simulink model "SimulinkModelisation"  (R2016b)
settings: Solver=VariableStepAuto  StartTime=0.0  StopTime=10.0  RelTol=1e-3  EnableMultiTasking=on
values from neighbouring files (symbols this model uses):
  A = [line1;line2;line3;line4;line5]    [sm_7.m]
  B = [m0_3x3; m0_3x3; m0_2x3; m0_2x3; mCV_3x3]    [sm_7.m]
  C = [mTTdef m0_3x3 m0_3x4 m0_3x3 ... (first row only)    [sm_7.m]
  D = zeros(7,3)    [sm_7.m]
undefined symbols (not defined in the file or in its folder): ae0, ae1, ae2, ae3, as0, as1, as2, as3, be1, C_prime, D_prime, ia_e, ib_e, ic_e, phi_e, TABC_trans, TDEF_trans, theta_e, va_e, vb_e, vc_e, vx_s_e, vy_s_e, vz_e, w_phi_e, w_theta_e, x_s_e, y_s_e, z_e, za_e, zb_e, zc_e, zd_e, ze_e, zf_e
settings Model: Creator=JayMcGee  LastModifiedBy=Sytten
settings OptimizationCC: LifeSpan=inf
settings DebuggingCC: SFUnexpectedBacktrackingDiag=warning  SFNoUnconditionalDefaultTransitionDiag=warning  SFExecutionAtInitializationDiag=none
settings GRTTargetCC: TargetLangStandard=C89/C90 (ANSI)  GeneratePreprocessorConditionals=Disable all
settings ConfigComp: CovMetricSettings=dw  CovHtmlReporting=on  CovSaveCumulativeToWorkspaceVar=on  CovSaveSingleToWorkspaceVar=on  CovExternalEMLEnable=off

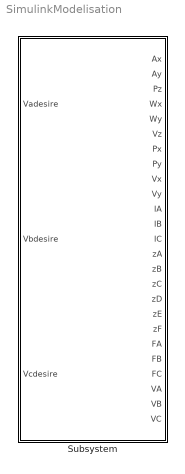
== system SimulinkModelisation ==
  Subsystem : Subsystem

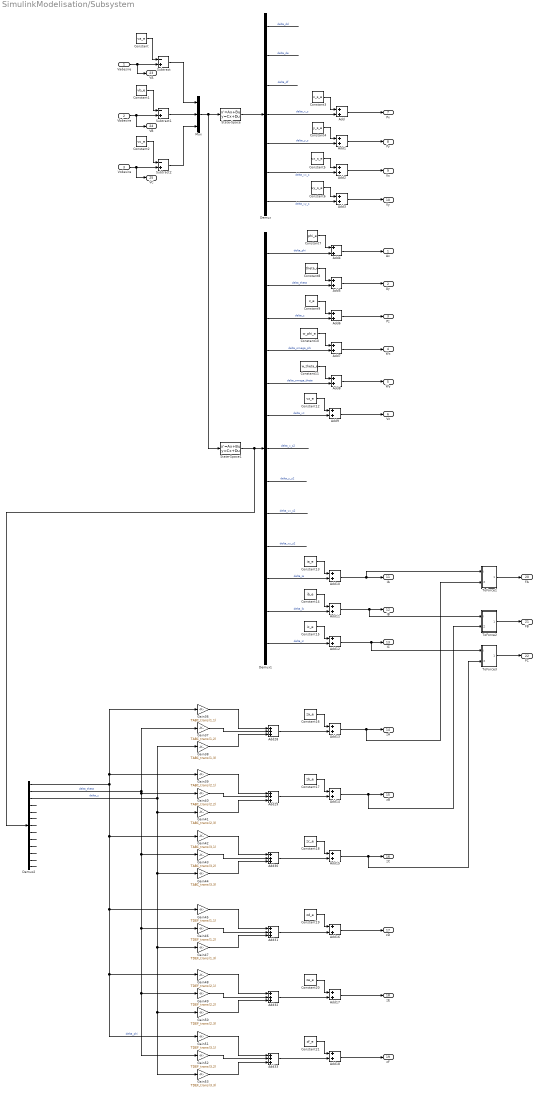
== system SimulinkModelisation/Subsystem ==
  Vadesire : Inport
  Vbdesire : Inport  Port=2
  Vcdesire : Inport  Port=3
  Add{,1..18} (19 alike) : Sum
  Add{28..33} (6 alike) : Sum  Inputs=+++
  Constant : Constant  Value=va_e
  Constant1 : Constant  Value=vb_e
  Constant10 : Constant  Value=w_phi_e
  Constant11 : Constant  Value=w_theta_e
  Constant12 : Constant  Value=vz_e
  Constant13 : Constant  Value=ia_e
  Constant14 : Constant  Value=ib_e
  Constant15 : Constant  Value=ic_e
  Constant16 : Constant  Value=za_e
  Constant17 : Constant  Value=zb_e
  Constant18 : Constant  Value=zc_e
  Constant19 : Constant  Value=zd_e
  Constant2 : Constant  Value=vc_e
  Constant20 : Constant  Value=ze_e
  Constant21 : Constant  Value=zf_e
  Constant3 : Constant  Value=x_s_e
  Constant4 : Constant  Value=y_s_e
  Constant5 : Constant  Value=vx_s_e
  Constant6 : Constant  Value=vy_s_e
  Constant7 : Constant  Value=phi_e
  Constant8 : Constant  Value=theta_e
  Constant9 : Constant  Value=z_e
  Demux : Demux  Outputs=7
  Demux1 : Demux  Outputs=13
  Demux2 : Demux  Outputs=13
  Gain36 : Gain  Gain=TABC_trans(1,1)
  Gain37 : Gain  Gain=TABC_trans(1,2)
  Gain38 : Gain  Gain=TABC_trans(1,3)
  Gain39 : Gain  Gain=TABC_trans(2,1)
  Gain40 : Gain  Gain=TABC_trans(2,2)
  Gain41 : Gain  Gain=TABC_trans(2,3)
  Gain42 : Gain  Gain=TABC_trans(3,1)
  Gain43 : Gain  Gain=TABC_trans(3,2)
  Gain44 : Gain  Gain=TABC_trans(3,3)
  Gain45 : Gain  Gain=TDEF_trans(1,1)
  Gain46 : Gain  Gain=TDEF_trans(1,2)
  Gain47 : Gain  Gain=TDEF_trans(1,3)
  Gain48 : Gain  Gain=TDEF_trans(2,1)
  Gain49 : Gain  Gain=TDEF_trans(2,2)
  Gain50 : Gain  Gain=TDEF_trans(2,3)
  Gain51 : Gain  Gain=TDEF_trans(3,1)
  Gain52 : Gain  Gain=TDEF_trans(3,2)
  Gain53 : Gain  Gain=TDEF_trans(3,3)
  Mux : Mux  Inputs=3
  State-Space : StateSpace  A=A  B=B  C=C  D=D  X0=0
  State-Space1 : StateSpace  A=A  B=B  C=C_prime  D=D_prime  X0=0
  Subtract : Sum  Inputs=-+
  Subtract1 : Sum  Inputs=-+
  Subtract2 : Sum  Inputs=-+
  ToForce1 : Subsystem
  ToForce2 : Subsystem
  ToForce3 : Subsystem
  Ax : Outport
  Ay : Outport  Port=2
  Pz : Outport  Port=3
  Wx : Outport  Port=4
  Wy : Outport  Port=5
  Vz : Outport  Port=6
  Px : Outport  Port=7
  Py : Outport  Port=8
  Vx : Outport  Port=9
  Vy : Outport  Port=10
  IA : Outport  Port=11
  IB : Outport  Port=12
  IC : Outport  Port=13
  zA : Outport  Port=14
  zB : Outport  Port=15
  zC : Outport  Port=16
  zD : Outport  Port=17
  zE : Outport  Port=18
  zF : Outport  Port=19
  FA : Outport  Port=20
  FB : Outport  Port=21
  FC : Outport  Port=22
  VA : Outport  Port=23
  VB : Outport  Port=24
  VC : Outport  Port=25
  wires:
  Demux2/6 -> ?
  Demux2/11 -> ?
  Add11/1 -> ToForce2/1(I), IB/1
  Demux2/7 -> ?
  Demux2/13 -> ?
  Gain44/1 -> Add30/3
  Constant13/1 -> Add10/1
  Constant15/1 -> Add12/1
  Gain50/1 -> Add32/3
  Demux1/13 -> Add12/2  "delta_ic"
  Demux1/7 -> ?  "delta_x_s2"
  Gain52/1 -> Add33/2
  Gain36/1 -> Add28/1
  Constant14/1 -> Add11/1
  Demux2/1 -> Gain48/1, Gain51/1, Gain45/1, Gain42/1, Gain39/1, Gain36/1  "delta_phi"
  Gain38/1 -> Add28/3
  Demux2/2 -> Gain37/1, Gain40/1, Gain52/1, Gain49/1, Gain46/1, Gain43/1  "delta_theta"
  Constant18/1 -> Add15/1
  Add28/1 -> Add13/2
  Add29/1 -> Add14/2
  Demux1/1 -> Add4/2  "delta_phi"
  Gain39/1 -> Add29/1
  Constant16/1 -> Add13/1
  Add30/1 -> Add15/2
  Constant11/1 -> Add8/1
  Demux1/4 -> Add7/2  "delta_omega_phi"
  Add2/1 -> Vx/1
  State-Space1/1 -> Demux2/1, Demux1/1
  Constant1/1 -> Subtract1/1
  Add1/1 -> Py/1
  Demux/2 -> ?  "delta_de"
  Vadesire/1 -> VA/1, Subtract/2
  Add3/1 -> Vy/1
  Constant17/1 -> Add14/1
  Constant4/1 -> Add1/1
  Constant3/1 -> Add/1
  Demux/4 -> Add/2  "delta_x_s"
  Demux/3 -> ?  "delta_df"
  Add9/1 -> Vz/1
  Constant12/1 -> Add9/1
  Constant5/1 -> Add2/1
  Demux1/6 -> Add9/2  "delta_vz"
  Demux1/10 -> ?  "delta_vy_s2"
  Vcdesire/1 -> VC/1, Subtract2/2
  Subtract1/1 -> Mux/2
  Add8/1 -> Wy/1
  Constant2/1 -> Subtract2/1
  Constant6/1 -> Add3/1
  Subtract2/1 -> Mux/3
  Add16/1 -> zD/1
  Add17/1 -> zE/1
  State-Space/1 -> Demux/1
  Gain53/1 -> Add33/3
  Demux1/9 -> ?  "delta_vx_s2"
  Demux2/10 -> ?
  Add33/1 -> Add18/2
  Demux/1 -> ?  "delta_dd"
  Subtract/1 -> Mux/1
  Demux/5 -> Add1/2  "delta_y_s"
  Add13/1 -> ToForce1/2(Z), zA/1
  Gain48/1 -> Add32/1
  Gain51/1 -> Add33/1
  Add15/1 -> ToForce3/2(Z), zC/1
  Add7/1 -> Wx/1
  Gain47/1 -> Add31/3
  Add14/1 -> ToForce2/2(Z), zB/1
  Constant10/1 -> Add7/1
  Add18/1 -> zF/1
  Gain43/1 -> Add30/2
  Demux2/3 -> Gain53/1, Gain50/1, Gain47/1, Gain44/1, Gain41/1, Gain38/1  "delta_z"
  Constant/1 -> Subtract/1
  Constant19/1 -> Add16/1
  Add32/1 -> Add17/2
  Add31/1 -> Add16/2
  Gain42/1 -> Add30/1
  Gain41/1 -> Add29/3
  Demux1/2 -> Add5/2  "delta_theta"
  Gain49/1 -> Add32/2
  Mux/1 -> State-Space1/1, State-Space/1
  Demux1/8 -> ?  "delta_y_s2"
  Demux/7 -> Add3/2  "delta_vy_s"
  Constant20/1 -> Add17/1
  Gain40/1 -> Add29/2
  Demux1/5 -> Add8/2  "delta_omega_theta"
  Demux2/4 -> ?
  Demux2/9 -> ?
  Demux2/8 -> ?
  Demux2/5 -> ?
  Demux1/12 -> Add11/2  "delta_ib"
  Vbdesire/1 -> VB/1, Subtract1/2
  Add/1 -> Px/1
  Demux/6 -> Add2/2  "delta_vx_s"
  Gain37/1 -> Add28/2
  Constant7/1 -> Add4/1
  Constant9/1 -> Add6/1
  Add5/1 -> Ay/1
  Add12/1 -> ToForce3/1(I), IC/1
  Demux1/3 -> Add6/2  "delta_z"
  Add6/1 -> Pz/1
  Constant8/1 -> Add5/1
  Gain46/1 -> Add31/2
  Demux1/11 -> Add10/2  "delta_ia"
  Gain45/1 -> Add31/1
  Add4/1 -> Ax/1
  Add10/1 -> ToForce1/1(I), IA/1
  Constant21/1 -> Add18/1
  Demux2/12 -> ?
  ToForce1/1(Force) -> FA/1
  ToForce2/1(Force) -> FB/1
  ToForce3/1(Force) -> FC/1

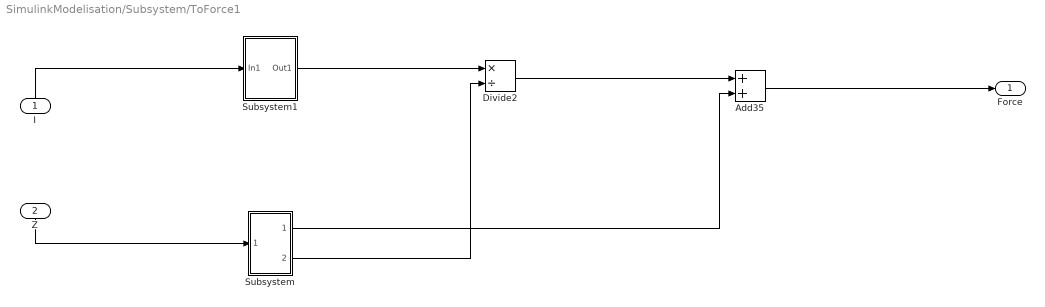
== system SimulinkModelisation/Subsystem/ToForce1 ==
  I : Inport
  Z : Inport  Port=2
  Add35 : Sum
  Divide2 : Product  Inputs=*/
  Subsystem : Subsystem
  Subsystem1 : Subsystem
  Force : Outport
  wires:
  Subsystem1/1(Out1) -> Divide2/1
  Z/1 -> Subsystem/1(In1)
  Subsystem/2(Out2) -> Divide2/2
  Divide2/1 -> Add35/1
  Add35/1 -> Force/1
  I/1 -> Subsystem1/1(In1)
  Subsystem/1(Out1) -> Add35/2

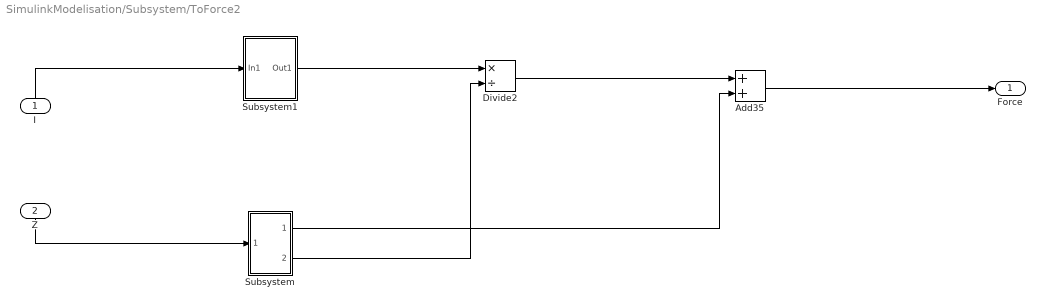
== system SimulinkModelisation/Subsystem/ToForce2 ==
  I : Inport
  Z : Inport  Port=2
  Add35 : Sum
  Divide2 : Product  Inputs=*/
  Subsystem : Subsystem
  Subsystem1 : Subsystem
  Force : Outport
  wires:
  Subsystem1/1(Out1) -> Divide2/1
  Z/1 -> Subsystem/1(In1)
  Subsystem/2(Out2) -> Divide2/2
  Divide2/1 -> Add35/1
  Add35/1 -> Force/1
  I/1 -> Subsystem1/1(In1)
  Subsystem/1(Out1) -> Add35/2

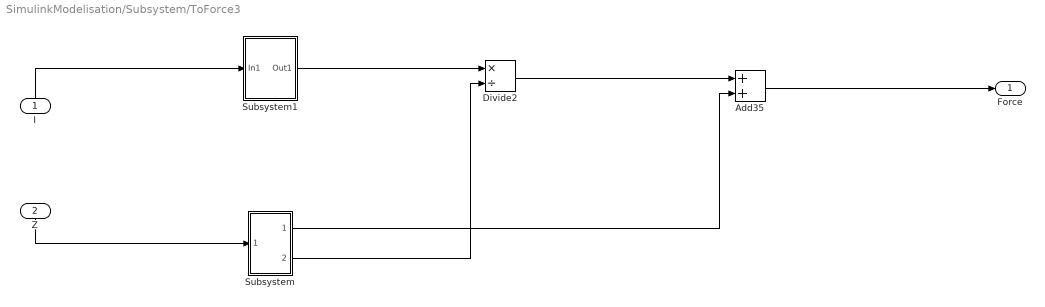
== system SimulinkModelisation/Subsystem/ToForce3 ==
  I : Inport
  Z : Inport  Port=2
  Add35 : Sum
  Divide2 : Product  Inputs=*/
  Subsystem : Subsystem
  Subsystem1 : Subsystem
  Force : Outport
  wires:
  Subsystem1/1(Out1) -> Divide2/1
  Z/1 -> Subsystem/1(In1)
  Subsystem/2(Out2) -> Divide2/2
  Divide2/1 -> Add35/1
  Add35/1 -> Force/1
  I/1 -> Subsystem1/1(In1)
  Subsystem/1(Out1) -> Add35/2

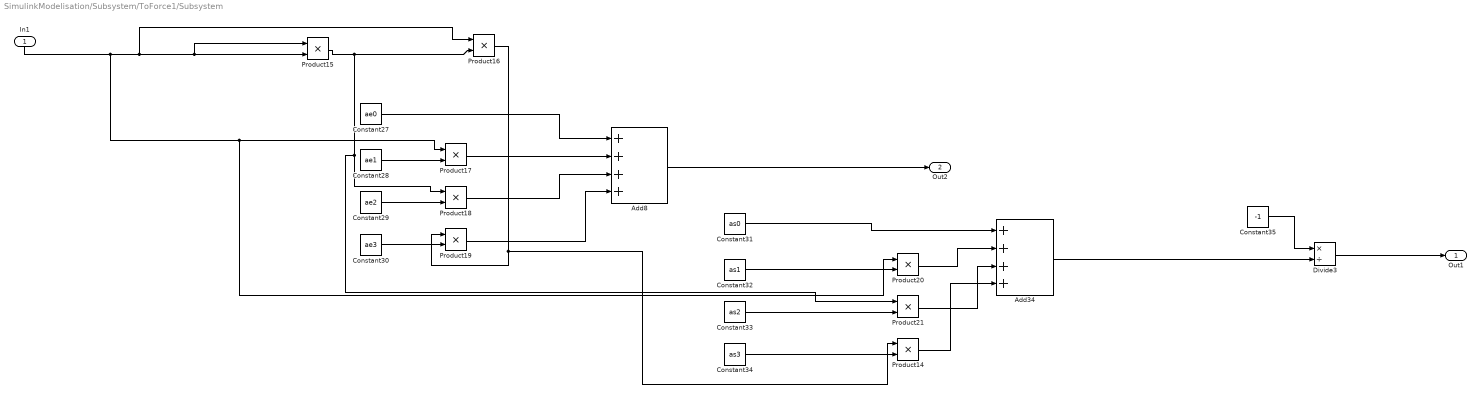
== system SimulinkModelisation/Subsystem/ToForce1/Subsystem ==
  In1 : Inport
  Add34 : Sum  Inputs=++++
  Add8 : Sum  Inputs=++++
  Constant27 : Constant  Value=ae0
  Constant28 : Constant  Value=ae1
  Constant29 : Constant  Value=ae2
  Constant30 : Constant  Value=ae3
  Constant31 : Constant  Value=as0
  Constant32 : Constant  Value=as1
  Constant33 : Constant  Value=as2
  Constant34 : Constant  Value=as3
  Constant35 : Constant  Value=-1
  Divide3 : Product  Inputs=*/
  Product{14..21} (8 alike) : Product
  Out1 : Outport
  Out2 : Outport  Port=2
  wires:
  In1/1 -> Product20/1, Product17/1, Product16/1, Product15/1, Product15/2
  Constant28/1 -> Product17/2
  Constant30/1 -> Product19/2
  Constant29/1 -> Product18/2
  Product15/1 -> Product21/1, Product18/1, Product16/2
  Product16/1 -> Product19/1, Product14/1
  Constant27/1 -> Add8/1
  Product17/1 -> Add8/2
  Product18/1 -> Add8/3
  Product19/1 -> Add8/4
  Add8/1 -> Out2/1
  Constant34/1 -> Product14/2
  Constant32/1 -> Product20/2
  Constant33/1 -> Product21/2
  Product20/1 -> Add34/2
  Product21/1 -> Add34/3
  Product14/1 -> Add34/4
  Constant31/1 -> Add34/1
  Add34/1 -> Divide3/2
  Constant35/1 -> Divide3/1
  Divide3/1 -> Out1/1

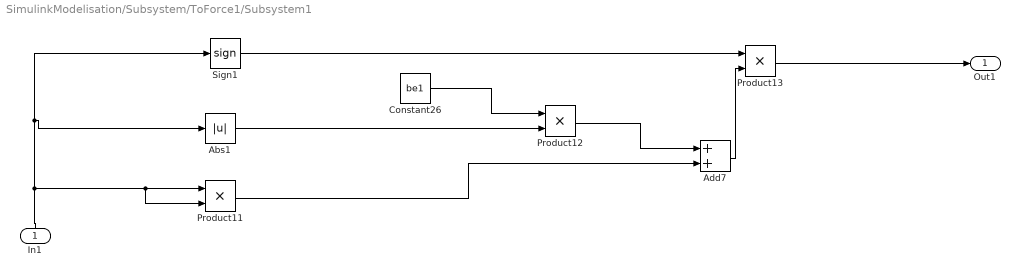
== system SimulinkModelisation/Subsystem/ToForce1/Subsystem1 ==
  In1 : Inport
  Abs1 : Abs
  Add7 : Sum
  Constant26 : Constant  Value=be1
  Product11 : Product
  Product12 : Product
  Product13 : Product
  Sign1 : Signum
  Out1 : Outport
  wires:
  In1/1 -> Abs1/1, Sign1/1, Product11/2, Product11/1
  Constant26/1 -> Product12/1
  Abs1/1 -> Product12/2
  Product12/1 -> Add7/1
  Product11/1 -> Add7/2
  Add7/1 -> Product13/2
  Product13/1 -> Out1/1
  Sign1/1 -> Product13/1

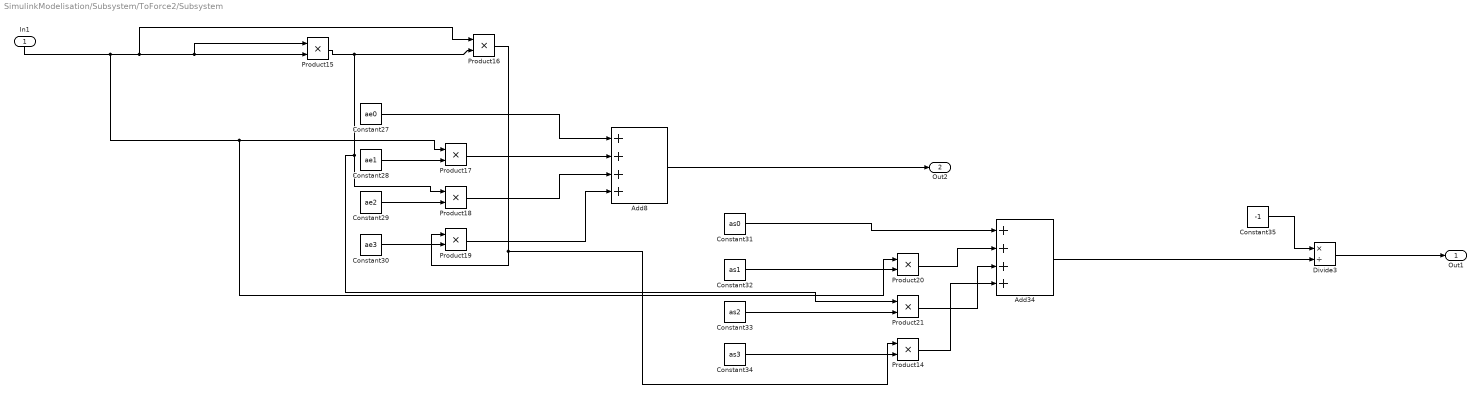
== system SimulinkModelisation/Subsystem/ToForce2/Subsystem ==
  In1 : Inport
  Add34 : Sum  Inputs=++++
  Add8 : Sum  Inputs=++++
  Constant27 : Constant  Value=ae0
  Constant28 : Constant  Value=ae1
  Constant29 : Constant  Value=ae2
  Constant30 : Constant  Value=ae3
  Constant31 : Constant  Value=as0
  Constant32 : Constant  Value=as1
  Constant33 : Constant  Value=as2
  Constant34 : Constant  Value=as3
  Constant35 : Constant  Value=-1
  Divide3 : Product  Inputs=*/
  Product{14..21} (8 alike) : Product
  Out1 : Outport
  Out2 : Outport  Port=2
  wires:
  In1/1 -> Product20/1, Product17/1, Product16/1, Product15/1, Product15/2
  Constant28/1 -> Product17/2
  Constant30/1 -> Product19/2
  Constant29/1 -> Product18/2
  Product15/1 -> Product21/1, Product18/1, Product16/2
  Product16/1 -> Product19/1, Product14/1
  Constant27/1 -> Add8/1
  Product17/1 -> Add8/2
  Product18/1 -> Add8/3
  Product19/1 -> Add8/4
  Add8/1 -> Out2/1
  Constant34/1 -> Product14/2
  Constant32/1 -> Product20/2
  Constant33/1 -> Product21/2
  Product20/1 -> Add34/2
  Product21/1 -> Add34/3
  Product14/1 -> Add34/4
  Constant31/1 -> Add34/1
  Add34/1 -> Divide3/2
  Constant35/1 -> Divide3/1
  Divide3/1 -> Out1/1

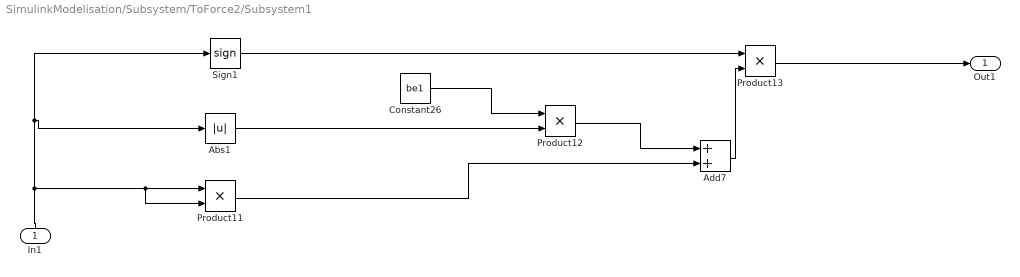
== system SimulinkModelisation/Subsystem/ToForce2/Subsystem1 ==
  In1 : Inport
  Abs1 : Abs
  Add7 : Sum
  Constant26 : Constant  Value=be1
  Product11 : Product
  Product12 : Product
  Product13 : Product
  Sign1 : Signum
  Out1 : Outport
  wires:
  In1/1 -> Abs1/1, Sign1/1, Product11/2, Product11/1
  Constant26/1 -> Product12/1
  Abs1/1 -> Product12/2
  Product12/1 -> Add7/1
  Product11/1 -> Add7/2
  Add7/1 -> Product13/2
  Product13/1 -> Out1/1
  Sign1/1 -> Product13/1

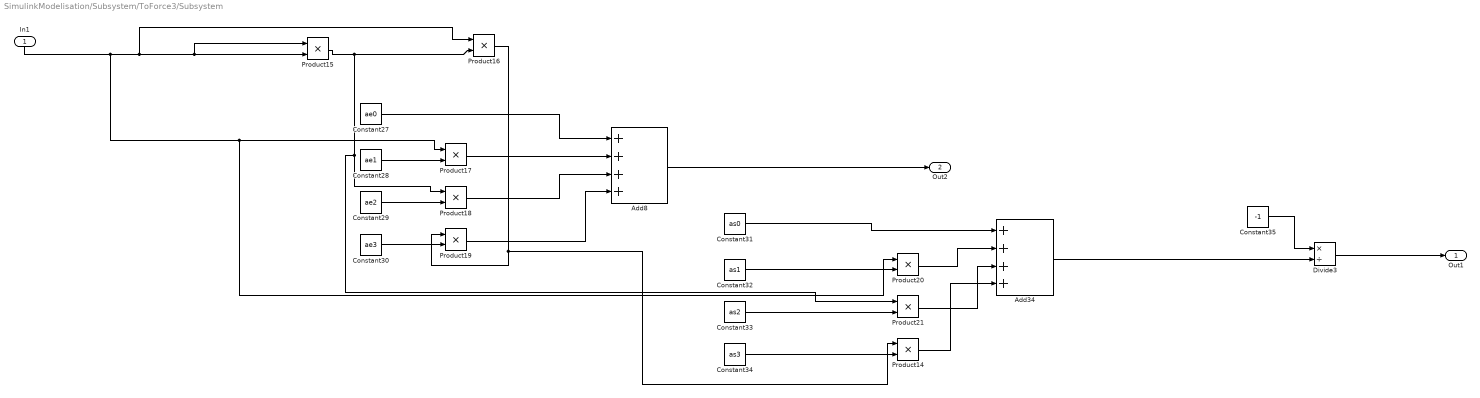
== system SimulinkModelisation/Subsystem/ToForce3/Subsystem ==
  In1 : Inport
  Add34 : Sum  Inputs=++++
  Add8 : Sum  Inputs=++++
  Constant27 : Constant  Value=ae0
  Constant28 : Constant  Value=ae1
  Constant29 : Constant  Value=ae2
  Constant30 : Constant  Value=ae3
  Constant31 : Constant  Value=as0
  Constant32 : Constant  Value=as1
  Constant33 : Constant  Value=as2
  Constant34 : Constant  Value=as3
  Constant35 : Constant  Value=-1
  Divide3 : Product  Inputs=*/
  Product{14..21} (8 alike) : Product
  Out1 : Outport
  Out2 : Outport  Port=2
  wires:
  In1/1 -> Product20/1, Product17/1, Product16/1, Product15/1, Product15/2
  Constant28/1 -> Product17/2
  Constant30/1 -> Product19/2
  Constant29/1 -> Product18/2
  Product15/1 -> Product21/1, Product18/1, Product16/2
  Product16/1 -> Product19/1, Product14/1
  Constant27/1 -> Add8/1
  Product17/1 -> Add8/2
  Product18/1 -> Add8/3
  Product19/1 -> Add8/4
  Add8/1 -> Out2/1
  Constant34/1 -> Product14/2
  Constant32/1 -> Product20/2
  Constant33/1 -> Product21/2
  Product20/1 -> Add34/2
  Product21/1 -> Add34/3
  Product14/1 -> Add34/4
  Constant31/1 -> Add34/1
  Add34/1 -> Divide3/2
  Constant35/1 -> Divide3/1
  Divide3/1 -> Out1/1

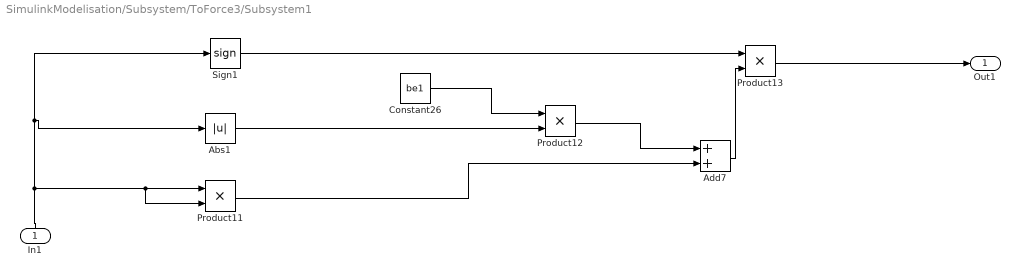
== system SimulinkModelisation/Subsystem/ToForce3/Subsystem1 ==
  In1 : Inport
  Abs1 : Abs
  Add7 : Sum
  Constant26 : Constant  Value=be1
  Product11 : Product
  Product12 : Product
  Product13 : Product
  Sign1 : Signum
  Out1 : Outport
  wires:
  In1/1 -> Abs1/1, Sign1/1, Product11/2, Product11/1
  Constant26/1 -> Product12/1
  Abs1/1 -> Product12/2
  Product12/1 -> Add7/1
  Product11/1 -> Add7/2
  Add7/1 -> Product13/2
  Product13/1 -> Out1/1
  Sign1/1 -> Product13/1
